simulink model "verify_HeatPump_CONF_mdl"  (R2016b)
settings: Solver=ode45  StartTime=0  StopTime=3600  MaxStep=600  RelTol=1e-3  EnableMultiTasking=on
InitFcn:
  | load('DE_TRY2010_13_averageYear')
undefined symbols (not defined in the file or in its folder): path_carnot
libraries: carnot x3
settings Model: Creator=drhf  LastModifiedBy=drhf
settings DataIOCC: SaveFormat=Array  SignalLoggingSaveFormat=ModelDataLogs
settings OptimizationCC: ExpressionDepthLimit=2147483647  LifeSpan=inf
settings DebuggingCC: UnderspecifiedInitializationDetection=Classic  MergeDetectMultiDrivingBlocksExec=none  SolverPrmCheckMsg=warning  FcnCallInpInsideContextMsg=warning  StateNameClashWarn=warning  SFUnexpectedBacktrackingDiag=warning  SFNoUnconditionalDefaultTransitionDiag=warning  SFExecutionAtInitializationDiag=none
settings HardwareCC: ProdBitPerPointer=32  ProdBitPerSizeT=32  ProdBitPerPtrDiffT=32  ProdLargestAtomicFloat=None  ProdIntDivRoundTo=Undefined  ProdEndianess=Unspecified  ProdWordSize=32  ProdHWDeviceType=32-bit Generic
settings ModelReferenceCC: PropagateSignalLabelsOutOfModel=off
settings GRTTargetCC: TargetLangStandard=C89/C90 (ANSI)  GeneratePreprocessorConditionals=Disable all  CombineOutputUpdateFcns=off  GRTInterface=on
settings ConfigComp: CovMetricSettings=dw  CovHtmlReporting=on  CovSaveCumulativeToWorkspaceVar=on  CovSaveSingleToWorkspaceVar=on  CovExternalEMLEnable=off

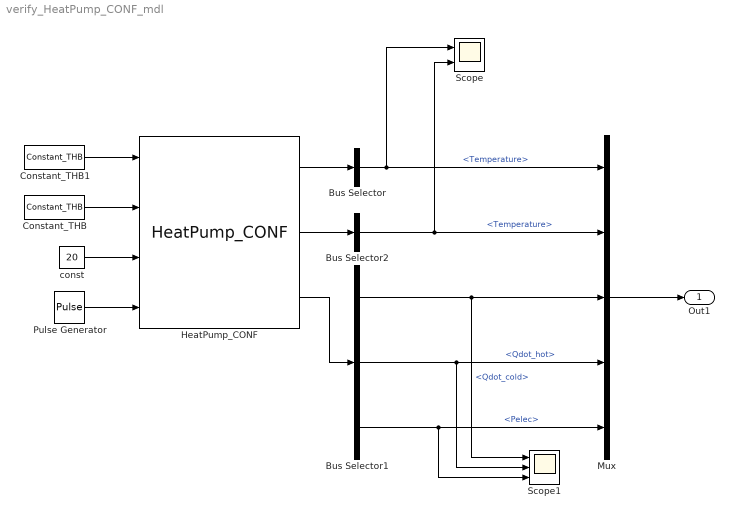
== system verify_HeatPump_CONF_mdl ==
  Bus Selector : BusSelector  OutputSignals=Temperature
  Bus Selector1 : BusSelector  OutputSignals=Qdot_cold,Qdot_hot,Pelec
  Bus Selector2 : BusSelector  OutputSignals=Temperature
  Constant_THB : carnot/Source/Simple/Constant_THB  t=40  mdot=2000/3600  p=1e5  mID=No Pressure Drop  fluid=Water  mix=0  mix2=0  mix3=0  dia=0.02  hgt=0
  Constant_THB1 : carnot/Source/Simple/Constant_THB  t=5  mdot=2000/3600  p=1e5  mID=No Pressure Drop  fluid=Water  mix=0  mix2=0  mix3=0  dia=0.02  hgt=0
  HeatPump_CONF : carnot/Source/Heat_Pump/HeatPump_CONF  PathName=fullfile(path_carnot('libsl'), 'Source','Heat_Pump','HeatPump_CONF','parameter_set')  FileName='DefaultHeatPump.mat'  userPath=off  userParam=off  K=[299.999998982327 -59.9999988176087 12249.9999711932 -6.66666603880034 60.0000010482174 -5.13158332307255e-05 306.666667839537 -115.000000230844 12225.0000010917]  caph=32000  capc=32000  UA=6  relQdotMin=1  linc=10  quac=100  linh=10  quah=100
  Mux : Mux  Inputs=5
  Pulse Generator : DiscretePulseGenerator  PulseType=Time based  Period=10*60  PulseWidth=50
  Scope : Scope  NumInputPorts=2
  Scope1 : Scope  NumInputPorts=3
  const : Constant  Value=20
  Out1 : Outport
  wires:
  HeatPump_CONF/1 -> Bus Selector/1
  Constant_THB/1 -> HeatPump_CONF/2
  Bus Selector/1 -> Mux/1, Scope/1  "<Temperature>"
  HeatPump_CONF/2 -> Bus Selector2/1
  const/1 -> HeatPump_CONF/3
  Pulse Generator/1 -> HeatPump_CONF/4
  Constant_THB1/1 -> HeatPump_CONF/1
  HeatPump_CONF/3 -> Bus Selector1/1
  Bus Selector2/1 -> Mux/2, Scope/2  "<Temperature>"
  Bus Selector1/3 -> Mux/5, Scope1/3  "<Pelec>"
  Bus Selector1/2 -> Mux/4, Scope1/2  "<Qdot_hot>"
  Bus Selector1/1 -> Mux/3, Scope1/1  "<Qdot_cold>"
  Mux/1 -> Out1/1
